simulink model "Detailed_PMSG_one_machine_GE"  (R2015b)
settings: Solver=VariableStepAuto  StartTime=0.0  StopTime=45  FixedStep=Ts  MaxStep=Ts  RelTol=1e-3
PreLoadFcn:
  | Ts=5e-6;
InitFcn:
  | Ts=5e-6;
undefined symbols (not defined in the file or in its folder): DiscIntNeverNeededParam, level
libraries: powerlib_extras x37, powerlib x16, simulink_extras x4, simulink x4
(part 1 of 2)
Description:
  | Copyright 2013-2015 Ruan Jiayang, Tsinghua Univ.
settings Model: Creator=XiaoLei  LastModifiedBy=Eren
settings DataIOCC: InitialState=xInit  SaveFinalState=on  SaveFormat=StructureWithTime  SignalLoggingSaveFormat=ModelDataLogs  SaveOutput=off  SignalLogging=off  SaveTime=off
settings OptimizationCC: ExpressionDepthLimit=2147483647  InitFltsAndDblsToZero=on
settings DebuggingCC: SaveWithParameterizedLinksMsg=none  UnderspecifiedInitializationDetection=Classic  MergeDetectMultiDrivingBlocksExec=none  SignalResolutionControl=TryResolveAllWithWarning  SolverPrmCheckMsg=warning  MultiTaskDSMMsg=warning  MultiTaskCondExecSysMsg=none  FcnCallInpInsideContextMsg=UseLocalSettings  UnconnectedInputMsg=none  UnconnectedOutputMsg=none  UnconnectedLineMsg=none  StateNameClashWarn=warning
settings HardwareCC: ProdBitPerPointer=32  ProdLargestAtomicFloat=None  ProdIntDivRoundTo=Undefined  ProdEndianess=Unspecified  ProdWordSize=32  ProdHWDeviceType=32-bit Generic
settings GRTTargetCC: TargetFcnLib=ansi_tfl_tmw.mat  GeneratePreprocessorConditionals=Disable all  CombineOutputUpdateFcns=off  GRTInterface=on
settings ConfigComp: CovModelRefEnable=Off

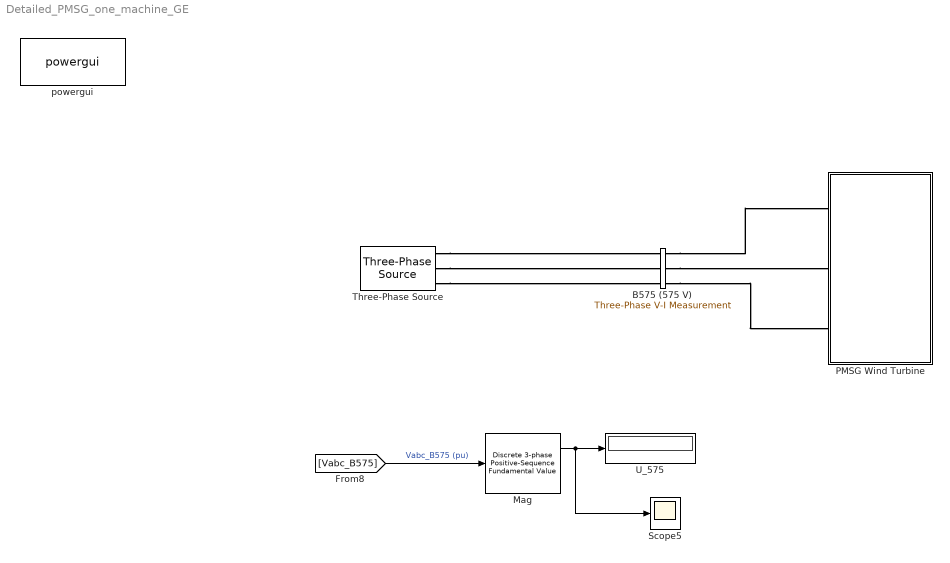
== system Detailed_PMSG_one_machine_GE ==
  B575 (575 V) : powerlib/Measurements/Three-Phase V-I Measurement  VoltageMeasurement=phase-to-ground  SetLabelV=on  LabelV=Vabc_B575  Vpu=on  VpuLL=off  CurrentMeasurement=yes  SetLabelI=on  LabelI=Iabc_B575  Ipu=on  Pbase=1.5e6  Vbase=575  OutputType=Complex  PhasorSimulation=off  PSBequivalent=0
  Mag : powerlib_extras/Discrete Measurements/Discrete 3-phase Positive-Sequence Fundamental Value  Freq=60  Par_Init=[0 0]  Ts=Ts
  PMSG Wind Turbine : Subsystem  mask{Vnom=575, Pnom=2.75e6, Fnom=50, RL_grid=[0.003 0.3], Vdc_nom=1150, Np=2, Fb_time_const=0.005}
      mask prompts: Vnom "Rated L-L Voltage(V)"; Pnom "Rated Power(VA)"; Fnom "Rated Frequency(Hz)"; RL_grid "Grid-side coupling impedance(p.u.)"; Vdc_nom "DC capacitor voltage(V)"; Np "Number of pole pairs"; Fb_time_const "Feed back time constant(s)"
      mask init:
      | R_RL=RL_grid(1);
      | L_RL=RL_grid(2);
  Scope5 : Scope
  Three-Phase Source : powerlib/Electrical Sources/Three-Phase Source  InternalConnection=Yg  VoltagePhases=off  Voltage=575  PhaseAngle=0  Voltage_phases=[25e3 25e3 25e3]/sqrt(3)  PhaseAngles_phases=[0 -120 +120]  Frequency=50  NonIdealSource=on  SpecifyImpedance=off  Resistance=0.0001  Inductance=16.58e-6  ShortCircuitLevel=100e6  BaseVoltage=575  XRratio=7  BusType=swing  Pref=10e3  Qref=0  Prefabc=[10e3, 10e3, 10e3]  Qrefabc=[0, 0, 0]  Qmin=-inf  Qmax=inf
  U_575 : Display
      settings: Decimation=10000
  powergui : powerlib/powergui  SimulationMode=Discrete  SolverType=Tustin/Backward Euler (TBE)  SampleTime=Ts  frequency=50  SPID=off  DisableSnubberDevices=off  DisableRonSwitches=off  DisableVfSwitches=off  SwTol=0  DisplayEquations=off  Interpol=off  ExternalGateDelay=off  methode=off  Ts=0  FunctionMessages=off  echomessages=off  HookPort=off  EnableUseOfTLC=off  x0status=blocks  frequencyindice=0  Pbase=100e6  ErrMax=1e-4  Iterations=50  UnitsV=kV  UnitsW=MW  buscounter=0  RestoreLinks=warning  ResistiveCurrentMeasurement=off  Frange=[0:2:500]  Ylog=off  Xlog=on  ShowGrid=off  save=off  variable=ZData  structure=0  ZoomFFT=on  StartTime=0.0  cycles=1  DisplayStyle=1  fundamental=60  FreqAxis=off  MaxFrequency=1000  frequencyindicesteady=1  RmsSteady=1  display=off
  wires:
  [Vabc_B575] -> Mag/1  "Vabc_B575 (pu)"
  Mag/1 -> U_575/1, Scope5/1
  connections:
  B575 (575 V)/RConn1 -- PMSG Wind Turbine/RConn1
  B575 (575 V)/RConn2 -- PMSG Wind Turbine/RConn2
  B575 (575 V)/RConn3 -- PMSG Wind Turbine/RConn3
  Three-Phase Source/RConn1 -- B575 (575 V)/LConn1
  Three-Phase Source/RConn2 -- B575 (575 V)/LConn2
  Three-Phase Source/RConn3 -- B575 (575 V)/LConn3

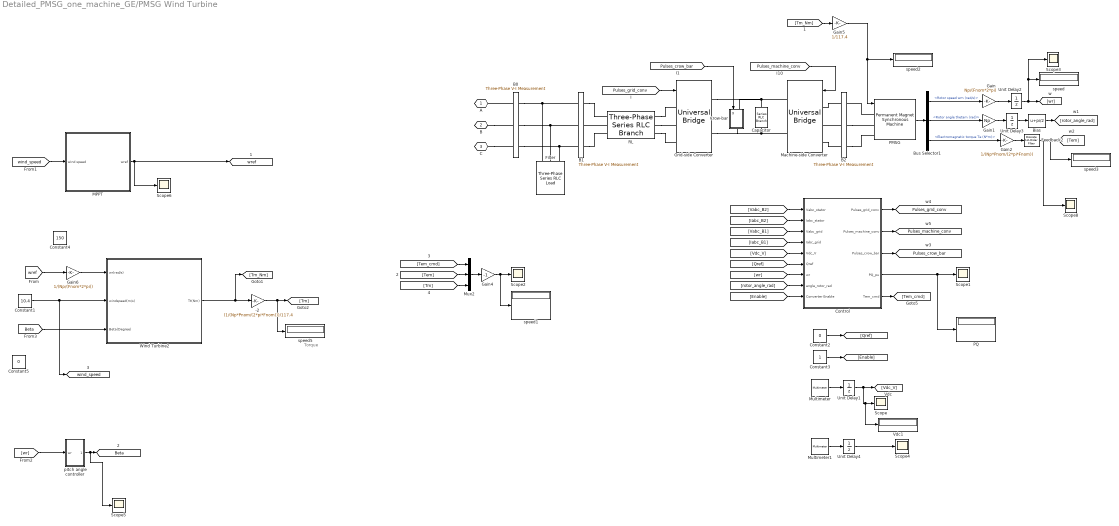
== system Detailed_PMSG_one_machine_GE/PMSG Wind Turbine ==
  note: Torque
  -2 : Gain  Gain=(1/(Np*Pnom/(2*pi*Fnom)))/117.4
  B0 : powerlib/Measurements/Three-Phase V-I Measurement  VoltageMeasurement=phase-to-ground  SetLabelV=on  LabelV=Vabc_B0  Vpu=on  VpuLL=off  CurrentMeasurement=yes  SetLabelI=on  LabelI=Iabc_B0  Ipu=on  Pbase=Pnom  Vbase=Vnom  OutputType=Complex  PhasorSimulation=off  PSBequivalent=0
  B1 : powerlib/Measurements/Three-Phase V-I Measurement  VoltageMeasurement=phase-to-ground  SetLabelV=on  LabelV=Vabc_B1  Vpu=on  VpuLL=off  CurrentMeasurement=yes  SetLabelI=on  LabelI=Iabc_B1  Ipu=on  Pbase=Pnom  Vbase=Vnom  OutputType=Complex  PhasorSimulation=off  PSBequivalent=0
  B2 : powerlib/Measurements/Three-Phase V-I Measurement  VoltageMeasurement=phase-to-ground  SetLabelV=on  LabelV=Vabc_B2  Vpu=on  VpuLL=off  CurrentMeasurement=yes  SetLabelI=on  LabelI=Iabc_B2  Ipu=on  Pbase=Pnom  Vbase=Vnom  OutputType=Complex  PhasorSimulation=off  PSBequivalent=0
  Bias : Bias  Bias=pi/2
  Bus Selector1 : BusSelector  OutputSignals=Rotor speed wm (rad/s),Rotor angle thetam (rad),Electromagnetic torque Te (N*m)
  Capacitor : powerlib/Elements/Series RLC Branch  LConnTagsString=__new0  RConnTagsString=__new0  BranchType=C  Resistance=1e-5  Inductance=1e-3  SetiL0=off  InitialCurrent=0  Capacitance=10000e-6  Setx0=on  InitialVoltage=Vdc_nom  Measurements=Branch voltage
  Constant1 : Constant  Value=10.4  SampleTime=Ts
  Constant2 : Constant  Value=0  SampleTime=Ts
  Constant3 : Constant  SampleTime=Ts
  Constant4 : Constant  Value=150  SampleTime=Ts
  Constant5 : Constant  Value=0  SampleTime=Ts
  Control : Subsystem
  Crow-bar : Subsystem
  Feedback2 : powerlib_extras/Discrete  Control Blocks/Discrete 1st-Order Filter  FilterType=Lowpass  Tc=0.3  Ts=Ts  Initialize=on  Vac_Init=[0 -25 60]  Vdc_Init=0  PlotResponse=off  param1=[1 500 0.1]
  Filter : powerlib/Elements/Three-Phase Series RLC Load  LConnTagsString=A|B|C  Configuration=Y (grounded)  NominalVoltage=Vnom  Vabc=[1e3 1e3 1e3]  Vabcp=[1e3 1e3 1e3]  NominalFrequency=Pnom  UnbalancedPower=off  ActivePower=0.005e6  InductivePower=0  CapacitivePower=0.04e6  Pabc=[10e3 9e3 11e3]  QLabc=[100 90 110]  QCabc=[100 90 110]  Pabcp=[10e3 9e3 11e3]  QLabcp=[100 90 110]  QCabcp=[100 90 110]  Measurements=None  LoadType=constant Z
  Gain : Gain  Gain=Np/(Fnom*2*pi)
  Gain1 : Gain  Gain=Np
  Gain2 : Gain  Gain=1/(Np*Pnom/(2*pi*Fnom))
  Gain4 : Gain  Gain=-1
  Gain5 : Gain  Gain=1/117.4
  Gain6 : Gain  Gain=1/(Np/(Fnom*2*pi))
  Grid-side Converter : powerlib/Power Electronics/Universal Bridge  Arms=3  SnubberResistance=1e5  SnubberCapacitance=inf  Device=IGBT / Diodes  Ron=1e-5  Lon=0  ForwardVoltages="[  0  0  ]"  ForwardVoltage=0  GTOparameters=[ 10e-6 , 20e-6 ]  IGBTparameters=[0 , 0]  Measurements=None  Measurements_2=None  converterType=Rectifier
  MPPT : Subsystem
  Machine-side Converter : powerlib/Power Electronics/Universal Bridge  Arms=3  SnubberResistance=1e5  SnubberCapacitance=inf  Device=IGBT / Diodes  Ron=1e-5  Lon=0  ForwardVoltages="[  0  0  ]"  ForwardVoltage=0  GTOparameters=[ 10e-6 , 20e-6 ]  IGBTparameters=[0 , 0]  Measurements=None  Measurements_2=None  converterType=Rectifier
  Multimeter : powerlib/Measurements/Multimeter  PhasorSimulation=off  OutputType=Complex  sel=1  L=2  Gain=1  yselected={'Ub: PMSG Wind Turbine/Capacitor'};  PSBOutputType=1  PSBequivalent=0  AxesSetting=[0,0.1,-100,100]  Display=0  SavedBlockNames=-11
  Multimeter1 : powerlib/Measurements/Multimeter  PhasorSimulation=off  OutputType=Complex  sel=2  L=2  Gain=1  yselected={'Ib: PMSG Wind Turbine/Crow-bar/R'};  PSBOutputType=1  PSBequivalent=0  AxesSetting=[0,0.1,-100,100]  Display=0  SavedBlockNames=-11
  Mux2 : Mux  Inputs=3
  PMSG : powerlib/Machines/Permanent Magnet Synchronous Machine  NbPhases=3  FluxDistribution=Sinusoidal  RotorType=Salient-pole  MechanicalLoad=Torque Tm  PresetModel=No  ShowDetailedParameters=on  MeasurementBus=off  Resistance=0.006  Inductance=8.5e-3  dqInductances="[2.48282e-4  2.92845e-4]"  La=2.48  MachineConstant=Flux linkage established by magnets (V.s)  Flux=4  VoltageCst=1451.0395  TorqueCst=12  Flat=120  Mechanical=[1088 0.01 Np]  PolePairs=Np  InitialConditions=[100,0, 0,0]  InitialConditions5ph=[0 0 0 0 0 0]  TsPowergui=0  TsBlock=Ts  RefAngle=90 degrees behind phase A axis (modified Park)
  PQ : Display
      settings: Decimation=10000
  RL : powerlib/Elements/Three-Phase Series RLC Branch  LConnTagsString=A|B|C  RConnTagsString=A|B|C  BranchType=RL  Resistance=R_RL*Vnom^2/Pnom  Inductance=L_RL*Vnom^2/Pnom/(2*pi*Fnom)  Capacitance=1.0  Measurements=None
  Scope{,1..6,8} (8 alike) : Scope
  Unit Delay{1..4} (4 alike) : UnitDelay  SampleTime=Ts
  Vdc1 : Display
      settings: Decimation=10000
  Wind Turbine2 : Subsystem
  pitch angle controller : Subsystem
  speed{,1..3,5} (5 alike) : Display
      speed settings: Decimation=10000
      speed1 settings: Decimation=10000
      speed2 settings: Decimation=1000
      speed3 settings: Decimation=1000
      speed5 settings: Decimation=1000
  A : PMIOPort  Tag=PMCPort  Port=1  Side=Right
  B : PMIOPort  Tag=PMCPort  Port=2  Side=Right
  C : PMIOPort  Tag=PMCPort  Port=3  Side=Right
  tag scope: Beta=global, Pulses_crow_bar=global, Pulses_grid_conv=global, Pulses_machine_conv=global, wind_speed=global, wref=global
  wires:
  Unit Delay1/1 -> [Vdc_V], Scope/1, Vdc1/1
  PMSG/1 -> Bus Selector1/1
  Bus Selector1/1 -> Gain/1  "<Rotor speed wm (rad/s)>"
  Gain/1 -> Unit Delay2/1
  Gain1/1 -> Unit Delay3/1
  Bus Selector1/2 -> Gain1/1  "<Rotor angle thetam (rad)>"
  Unit Delay2/1 -> [wr], speed/1, Scope3/1
  [Qref] -> Control/6(Qref)
  [Vdc_V] -> Control/5(Vdc_V)
  [Iabc_B1] -> Control/4(Iabc_grid)
  [Vabc_B1] -> Control/3(Vabc_grid)
  [Vabc_B2] -> Control/1(Vabc_stator)
  [Iabc_B2] -> Control/2(Iabc_stator)
  [Enable] -> Control/9(Converter Enable)
  Constant3/1 -> [Enable]
  Constant2/1 -> [Qref]
  [Pulses_grid_conv] -> Grid-side Converter/1
  [Pulses_machine_conv] -> Machine-side Converter/1
  Control/1(Pulses_grid_conv) -> [Pulses_grid_conv]
  Control/4(PQ_pu) -> Scope1/1, PQ/1
  Control/2(Pulses_machine_conv) -> [Pulses_machine_conv]
  [wr] -> Control/7(wr)
  [rotor_angle_rad] -> Control/8(angle_rotor_rad)
  Bus Selector1/3 -> Gain2/1  "<Electromagnetic torque Te (N*m)>"
  Bias/1 -> [rotor_angle_rad]
  Unit Delay3/1 -> Bias/1
  [Tm_Nm] -> Gain5/1
  Gain2/1 -> Feedback2/1
  Feedback2/1 -> Scope8/1, [Tem], speed3/1
  Control/5(Tem_cmd) -> [Tem_cmd]
  [Tem] -> Mux2/2
  [Tem_cmd] -> Mux2/1
  [Tm] -> Mux2/3
  Mux2/1 -> Gain4/1
  Gain4/1 -> Scope2/1, speed1/1
  Multimeter/1 -> Unit Delay1/1
  Control/3(Pulses_crow_bar) -> [Pulses_crow_bar]
  Unit Delay4/1 -> Scope4/1
  Multimeter1/1 -> Unit Delay4/1
  [Pulses_crow_bar] -> Crow-bar/1(g)
  [wr] -> pitch angle controller/1(wr)
  pitch angle controller/1(Beta) -> Scope5/1, [Beta]
  [wind_speed] -> MPPT/1(wind speed)
  MPPT/1("wref ") -> [wref], Scope6/1
  Gain5/1 -> speed2/1, PMSG/1
  -2/1 -> speed5/1, [Tm]
  Wind Turbine2/1(Tt(Nm)) -> [Tm_Nm], -2/1
  Constant1/1 -> [wind_speed], Wind Turbine2/2(windspeed(m/s))
  [wref] -> Gain6/1
  [Beta] -> Wind Turbine2/3(Beta(Degree))
  Gain6/1 -> Wind Turbine2/1(wr(rad/s))
  connections:
  RL/RConn1 -- Grid-side Converter/LConn1
  RL/RConn2 -- Grid-side Converter/LConn2
  RL/RConn3 -- Grid-side Converter/LConn3
  B1/LConn1 -- Filter/LConn1 -- B0/RConn1
  B1/LConn2 -- Filter/LConn2 -- B0/RConn2
  B1/LConn3 -- Filter/LConn3 -- B0/RConn3
  B1/RConn1 -- RL/LConn1
  RL/LConn2 -- B1/RConn2
  B1/RConn3 -- RL/LConn3
  B2/RConn2 -- PMSG/LConn2
  PMSG/LConn1 -- B2/RConn1
  B2/LConn1 -- Machine-side Converter/LConn1
  Machine-side Converter/LConn3 -- B2/LConn3
  B2/LConn2 -- Machine-side Converter/LConn2
  B0/LConn1 -- A/RConn1
  B/RConn1 -- B0/LConn2
  C/RConn1 -- B0/LConn3
  B2/RConn3 -- PMSG/LConn3
  Grid-side Converter/RConn1 -- Crow-bar/LConn1 -- Machine-side Converter/RConn1 -- Capacitor/LConn1
  Grid-side Converter/RConn2 -- Crow-bar/RConn1 -- Machine-side Converter/RConn2 -- Capacitor/RConn1

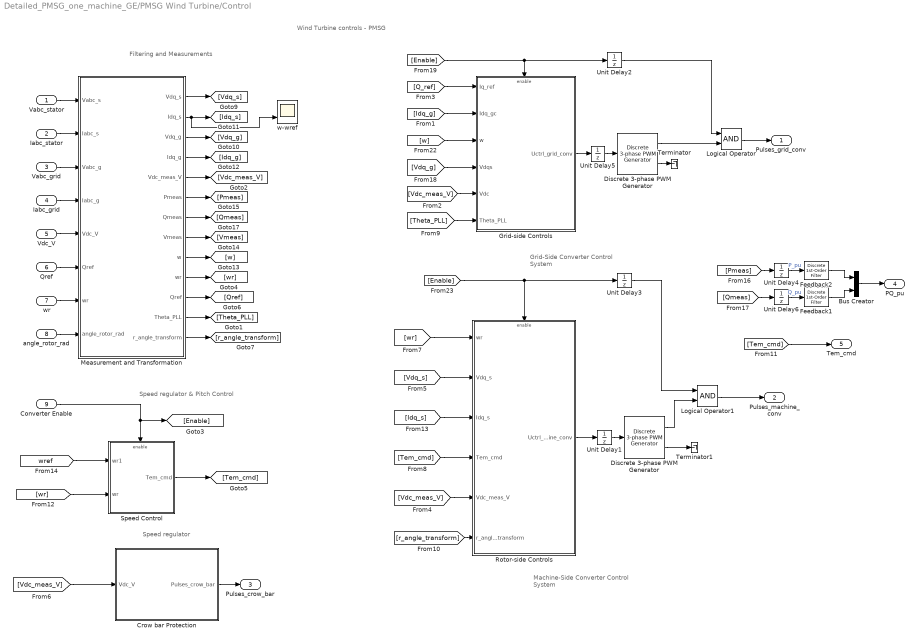
== system Detailed_PMSG_one_machine_GE/PMSG Wind Turbine/Control ==
  note: Wind Turbine controls - PMSG
  note: Filtering and
      | Measurements
  note: Speed regulator & Pitch Control
  note: Speed regulator
  note: Grid-Side Converter
      | Control System
  note: Machine-Side Converter
      | Control System
  Vabc_stator : Inport
  Iabc_stator : Inport  Port=2
  Vabc_grid : Inport  Port=3
  Iabc_grid : Inport  Port=4
  Vdc_V : Inport  Port=5
  Qref : Inport  Port=6
  wr : Inport  Port=7
  angle_rotor_rad : Inport  Port=8
  Converter Enable : Inport  Port=9
  Bus Creator : BusCreator  Inputs=2
  Crow bar Protection : Subsystem
  Discrete 3-phase PWM Generator : powerlib_extras/Discrete  Control Blocks/Discrete 3-phase PWM Generator  ModulatorType=2-level  ModulatorMode=Un-synchronized  nF=27  Fc=2250  ModulatingSignals=off  m=0.2  Freq=60  Phase=0  Ts=Ts
  "Discrete 3-phase PWM Generator " : powerlib_extras/Discrete  Control Blocks/Discrete 3-phase PWM Generator  ModulatorType=2-level  ModulatorMode=Un-synchronized  nF=27  Fc=3000  ModulatingSignals=off  m=0.2  Freq=60  Phase=0  Ts=Ts
  Feedback1 : powerlib_extras/Discrete  Control Blocks/Discrete 1st-Order Filter  FilterType=Lowpass  Tc=0.3  Ts=Ts  Initialize=on  Vac_Init=[0 -25 50]  Vdc_Init=0  PlotResponse=off  param1=[1 500 0.1]
  Feedback2 : powerlib_extras/Discrete  Control Blocks/Discrete 1st-Order Filter  FilterType=Lowpass  Tc=0.3  Ts=Ts  Initialize=on  Vac_Init=[0 -25 50]  Vdc_Init=0  PlotResponse=off  param1=[1 500 0.1]
  Grid-side Controls : Subsystem
  Logical Operator : Logic  AllPortsSameDT=off  OutDataTypeStr=boolean
  Logical Operator1 : Logic  AllPortsSameDT=off  OutDataTypeStr=boolean
  Measurement and Transformation : Subsystem
  Rotor-side Controls : Subsystem
  Speed Control : Subsystem
  Terminator : Terminator
  Terminator1 : Terminator
  Unit Delay{1..6} (6 alike) : UnitDelay  SampleTime=Ts
  w-wref : Scope  NumInputPorts=2
  Pulses_grid_conv : Outport
  Pulses_machine_conv : Outport  Port=2
  Pulses_crow_bar : Outport  Port=3
  PQ_pu : Outport  Port=4
  Tem_cmd : Outport  Port=5
  wires:
  [Pmeas] -> Unit Delay4/1
  [Qmeas] -> Unit Delay6/1
  wr/1 -> Measurement and Transformation/7(wr)
  Qref/1 -> Measurement and Transformation/6(Qref)
  Vdc_V/1 -> Measurement and Transformation/5(Vdc_V)
  Measurement and Transformation/11("Qref ") -> [Qref]
  Measurement and Transformation/10("wr ") -> [wr]
  Measurement and Transformation/5(Vdc_meas_V) -> [Vdc_meas_V]
  Measurement and Transformation/9(w) -> [w]
  Measurement and Transformation/6(Pmeas) -> [Pmeas]
  Measurement and Transformation/4(Idq_g) -> [Idq_g]
  Measurement and Transformation/3(Vdq_g) -> [Vdq_g]
  Measurement and Transformation/2(Idq_s) -> w-wref/2, [Idq_s]
  angle_rotor_rad/1 -> Measurement and Transformation/8(angle_rotor_rad)
  Iabc_stator/1 -> Measurement and Transformation/2(Iabc_s)
  Iabc_grid/1 -> Measurement and Transformation/4(Iabc_g)
  Vabc_grid/1 -> Measurement and Transformation/3(Vabc_g)
  Vabc_stator/1 -> Measurement and Transformation/1(Vabc_s)
  Measurement and Transformation/7(Qmeas) -> [Qmeas]
  Measurement and Transformation/8(Vmeas) -> [Vmeas]
  Measurement and Transformation/12(Theta_PLL) -> [Theta_PLL]
  Measurement and Transformation/13(r_angle_transform) -> [r_angle_transform]
  Speed Control/1(Tem_cmd) -> [Tem_cmd]
  [wr] -> Speed Control/2(wr)
  Converter Enable/1 -> Speed Control/Enable, [Enable]
  [Tem_cmd] -> Tem_cmd/1
  Measurement and Transformation/1(Vdq_s) -> [Vdq_s]
  Grid-side Controls/1(Uctrl_grid_conv) -> Unit Delay5/1
  Discrete 3-phase PWM Generator/2 -> Terminator/1
  Unit Delay5/1 -> Discrete 3-phase PWM Generator/1
  [Vdc_meas_V] -> Grid-side Controls/5(Vdc)
  [Vdq_g] -> Grid-side Controls/4(Vdqs)
  [w] -> Grid-side Controls/3(w)
  [Idq_g] -> Grid-side Controls/2(Idq_gc)
  [Q_ref] -> Grid-side Controls/1(Iq_ref)
  [Theta_PLL] -> Grid-side Controls/6(Theta_PLL)
  [Enable] -> Grid-side Controls/Enable, Unit Delay2/1
  Logical Operator/1 -> Pulses_grid_conv/1
  Discrete 3-phase PWM Generator/1 -> Logical Operator/2
  Unit Delay2/1 -> Logical Operator/1
  "Discrete 3-phase PWM Generator "/2 -> Terminator1/1
  Unit Delay1/1 -> "Discrete 3-phase PWM Generator "/1
  [Enable] -> Unit Delay3/1, Rotor-side Controls/Enable
  Logical Operator1/1 -> Pulses_machine_conv/1
  "Discrete 3-phase PWM Generator "/1 -> Logical Operator1/2
  Unit Delay3/1 -> Logical Operator1/1
  [wr] -> Rotor-side Controls/1(wr)
  [Vdc_meas_V] -> Rotor-side Controls/5(Vdc_meas_V)
  [r_angle_transform] -> Rotor-side Controls/6(r_angle_transform)
  [Vdq_s] -> Rotor-side Controls/2(" Vdq_s")
  [Idq_s] -> Rotor-side Controls/3(Idq_s)
  Rotor-side Controls/1(Uctrl_machine_conv) -> Unit Delay1/1
  [Tem_cmd] -> Rotor-side Controls/4(Tem_cmd)
  Unit Delay4/1 -> Feedback2/1  "P_pu"
  Feedback2/1 -> Bus Creator/1
  Unit Delay6/1 -> Feedback1/1  "Q_pu"
  Feedback1/1 -> Bus Creator/2
  Crow bar Protection/1(Pulses_crow_bar) -> Pulses_crow_bar/1
  [Vdc_meas_V] -> Crow bar Protection/1(Vdc_V)
  Bus Creator/1 -> PQ_pu/1
  [wref] -> Speed Control/1(wr1)

== system Detailed_PMSG_one_machine_GE/PMSG Wind Turbine/Crow-bar ==
  g : Inport
  IGBT : powerlib/Power Electronics/IGBT//Diode  Ron=1e-5  Rs=1e5  Cs=inf  Measurements=off
  R : powerlib/Elements/Series RLC Branch  LConnTagsString=__new0  RConnTagsString=__new0  BranchType=R  Resistance=1  Inductance=1e-3  SetiL0=off  InitialCurrent=0  Capacitance=1e-6  Setx0=off  InitialVoltage=0  Measurements=Branch current
  + : PMIOPort  Port=1  Side=Left
  - : PMIOPort  Port=2  Side=Right
  wires:
  g/1 -> IGBT/1
  connections:
  R/LConn1 -- IGBT/RConn1
  +/RConn1 -- IGBT/LConn1
  -/RConn1 -- R/RConn1

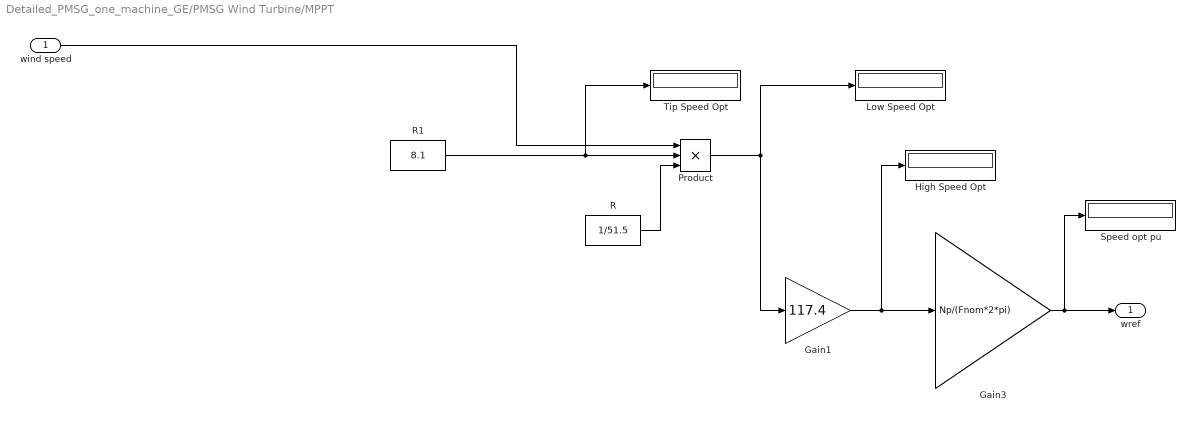
== system Detailed_PMSG_one_machine_GE/PMSG Wind Turbine/MPPT ==
  wind speed : Inport
  " High Speed Opt " : Display
  " Speed opt pu " : Display
  Gain1 : Gain  Gain=117.4
  Gain3 : Gain  Gain=Np/(Fnom*2*pi)
  "Low Speed Opt " : Display
  Product : Product  Inputs=3
  R : Constant  Value=1/51.5
  R1 : Constant  Value=8.1
  "Tip Speed Opt " : Display
  "wref " : Outport
  wires:
  R1/1 -> "Tip Speed Opt "/1, Product/2
  R/1 -> Product/3
  wind speed/1 -> Product/1
  Product/1 -> "Low Speed Opt "/1, Gain1/1
  Gain3/1 -> " Speed opt pu "/1, "wref "/1
  Gain1/1 -> " High Speed Opt "/1, Gain3/1

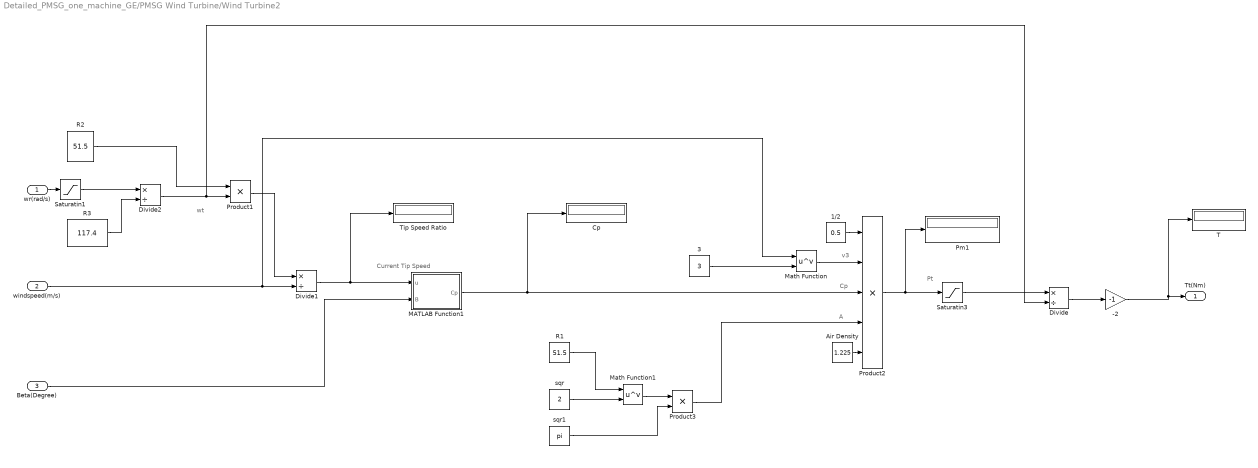
== system Detailed_PMSG_one_machine_GE/PMSG Wind Turbine/Wind Turbine2 ==
  note: Pt
  note: v3
  note: Cp
  note: A
  note: wt
  note: Current Tip Speed
  wr(rad/s) : Inport
  windspeed(m/s) : Inport  Port=2
  Beta(Degree) : Inport  Port=3
  -2 : Gain  Gain=-1
  1/2 : Constant  Value=0.5
  3 : Constant  Value=3
  Air Density : Constant  Value=1.225
  Cp : Display
  Divide : Product  Inputs=*/
  Divide1 : Product  Inputs=*/
  Divide2 : Product  Inputs=*/
  MATLAB Function1 : MATLAB Function  TreatAsAtomicUnit=on
  Math Function : Math  Operator=pow  SaturateOnIntegerOverflow=on
  Math Function1 : Math  Operator=pow  SaturateOnIntegerOverflow=on
  Pm1 : Display
  Product1 : Product
  Product2 : Product  Inputs=5
  Product3 : Product
  R1 : Constant  Value=51.5
  R2 : Constant  Value=51.5
  R3 : Constant  Value=117.4
  Saturatin1 : Saturate  UpperLimit=inf  LowerLimit=1e-8
  Saturatin3 : Saturate  UpperLimit=2.75e6  LowerLimit=1e-6
  T : Display
  "Tip Speed Ratio " : Display
  sqr : Constant  Value=2
  sqr1 : Constant  Value=pi
  Tt(Nm) : Outport
  wires:
  Air Density/1 -> Product2/5
  1/2/1 -> Product2/1
  Product3/1 -> Product2/4
  Math Function1/1 -> Product3/1
  sqr1/1 -> Product3/2
  Math Function/1 -> Product2/2
  sqr/1 -> Math Function1/2
  R1/1 -> Math Function1/1
  Product2/1 -> Saturatin3/1, Pm1/1
  3/1 -> Math Function/2
  R2/1 -> Product1/1
  wr(rad/s)/1 -> Saturatin1/1
  Product1/1 -> Divide1/1
  Divide1/1 -> MATLAB Function1/1(u), "Tip Speed Ratio "/1
  Divide2/1 -> Divide/2, Product1/2
  MATLAB Function1/1(Cp) -> Product2/3, Cp/1
  R3/1 -> Divide2/2
  windspeed(m/s)/1 -> Math Function/1, Divide1/2
  Beta(Degree)/1 -> MATLAB Function1/2(B)
  Divide/1 -> -2/1
  Saturatin3/1 -> Divide/1
  Saturatin1/1 -> Divide2/1
  -2/1 -> T/1, Tt(Nm)/1

== system Detailed_PMSG_one_machine_GE/PMSG Wind Turbine/pitch angle controller ==
  wr : Inport
  Constant1 : Constant  Value=1735/1500  SampleTime=Ts
  pitch angle controller : Subsystem
  Beta : Outport
  wires:
  Constant1/1 -> pitch angle controller/2(Ref)
  pitch angle controller/1(pitch) -> Beta/1
  wr/1 -> pitch angle controller/1(wg)

== system Detailed_PMSG_one_machine_GE/PMSG Wind Turbine/Control/Crow bar Protection ==
  Vdc_V : Inport
  Relay : Relay  OnSwitchValue=1500  OffSwitchValue=1300
  Pulses_crow_bar : Outport
  wires:
  Vdc_V/1 -> Relay/1
  Relay/1 -> Pulses_crow_bar/1

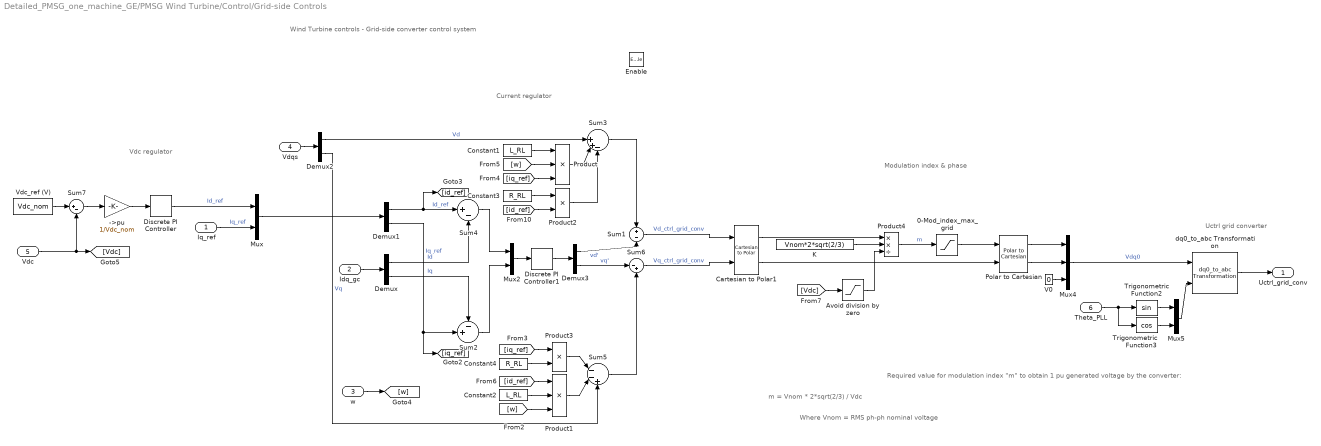
== system Detailed_PMSG_one_machine_GE/PMSG Wind Turbine/Control/Grid-side Controls ==
  note: Wind Turbine controls - Grid-side converter control system
  note: Where Vnom = RMS ph-ph nominal voltage
  note: m = Vnom * 2*sqrt(2/3) / Vdc
  note: Required value for modulation index "m" to obtain 1 pu generated voltage by the converter:
  note: Vdc regulator
  note: Current regulator
  note: Modulation index & phase
  note: Uctrl grid converter
  Iq_ref : Inport
  Idq_gc : Inport  Port=2
  w : Inport  Port=3
  Vdqs : Inport  Port=4
  Vdc : Inport  Port=5
  Theta_PLL : Inport  Port=6
  Enable : EnablePort
  ->pu : Gain  Gain=1/Vdc_nom
  0-Mod_index_max_grid : Saturate  UpperLimit=1.1  LowerLimit=0
  Avoid division by zero : Saturate  UpperLimit=inf  LowerLimit=1e-6
  Cartesian to Polar1 : simulink_extras/Transformations/Cartesian to Polar
  Constant1 : Constant  Value=L_RL
  Constant2 : Constant  Value=L_RL
  Constant3 : Constant  Value=R_RL
  Constant4 : Constant  Value=R_RL
  Demux{,1..3} (4 alike) : Demux  Outputs=2
  Discrete PI Controller : powerlib_extras/Discrete  Control Blocks/Discrete PI Controller  Kp=8  Ki=400  Par_Limits=[1 -1]*1.2  Init=0  Ts=Ts
  Discrete PI Controller1 : powerlib_extras/Discrete  Control Blocks/Discrete PI Controller  Kp=0.83  Ki=5  Par_Limits=[1.0 -1.0] *1.1  Init=0  Ts=Ts
  K : Constant  Value=Vnom*2*sqrt(2/3)
  Mux : Mux  Inputs=2
  Mux2 : Mux  Inputs=2
  Mux4 : Mux  Inputs=3
  Mux5 : Mux  Inputs=2
  Polar to Cartesian : simulink_extras/Transformations/Polar to Cartesian
  Product : Product  Inputs=3  SaturateOnIntegerOverflow=on  InputSameDT=on  OutDataTypeStr=Inherit: Same as first input
  Product1 : Product  Inputs=3  SaturateOnIntegerOverflow=on  InputSameDT=on  OutDataTypeStr=Inherit: Same as first input
  Product2 : Product  SaturateOnIntegerOverflow=on  InputSameDT=on  OutDataTypeStr=Inherit: Same as first input
  Product3 : Product  SaturateOnIntegerOverflow=on  InputSameDT=on  OutDataTypeStr=Inherit: Same as first input
  Product4 : Product  Inputs=**/  SaturateOnIntegerOverflow=on  InputSameDT=on  OutDataTypeStr=Inherit: Same as first input
  Sum1 : Sum  Inputs=+-  SaturateOnIntegerOverflow=on  InputSameDT=on  OutDataTypeStr=Inherit: Same as first input
  Sum2 : Sum  Inputs=-+|  SaturateOnIntegerOverflow=on  InputSameDT=on  OutDataTypeStr=Inherit: Same as first input
  Sum3 : Sum  Inputs=||++-  SaturateOnIntegerOverflow=on  InputSameDT=on  OutDataTypeStr=Inherit: Same as first input
  Sum4 : Sum  Inputs=|+-  SaturateOnIntegerOverflow=on  InputSameDT=on  OutDataTypeStr=Inherit: Same as first input
  Sum5 : Sum  Inputs=|--+  SaturateOnIntegerOverflow=on  InputSameDT=on  OutDataTypeStr=Inherit: Same as first input
  Sum6 : Sum  Inputs=|-+  SaturateOnIntegerOverflow=on  InputSameDT=on  OutDataTypeStr=Inherit: Same as first input
  Sum7 : Sum  Inputs=|+-  SaturateOnIntegerOverflow=on  InputSameDT=on  OutDataTypeStr=Inherit: Same as first input
  Trigonometric Function2 : Trigonometry
  Trigonometric Function3 : Trigonometry  Operator=cos
  V0 : Constant  Value=0
  Vdc_ref (V) : Constant  Value=Vdc_nom
  dq0_to_abc Transformation : powerlib_extras/Measurements/dq0_to_abc Transformation
  Uctrl_grid_conv : Outport
  wires:
  Vdc_ref (V)/1 -> Sum7/1
  Iq_ref/1 -> Mux/2  "Iq_ref"
  Vdc/1 -> Sum7/2, [Vdc]
  ->pu/1 -> Discrete PI Controller/1
  Sum7/1 -> ->pu/1
  Discrete PI Controller/1 -> Mux/1  "Id_ref"
  Sum5/1 -> Sum6/2
  Sum3/1 -> Sum1/1
  Demux1/1 -> [id_ref], Sum4/1  "Id_ref"
  Demux1/2 -> Sum2/2, [iq_ref]  "Iq_ref"
  Demux3/2 -> Sum6/1  "vq'"
  Demux3/1 -> Sum1/2  "vd'"
  [id_ref] -> Product1/1
  [iq_ref] -> Product3/1
  [id_ref] -> Product2/2
  [iq_ref] -> Product/3
  [w] -> Product/2
  [w] -> Product1/3
  Sum2/1 -> Mux2/2
  Sum4/1 -> Mux2/1
  Product3/1 -> Sum5/1
  Product2/1 -> Sum3/3
  Demux2/2 -> Sum5/3  "Vq"
  Product1/1 -> Sum5/2
  Constant4/1 -> Product3/2
  Constant3/1 -> Product2/1
  Product/1 -> Sum3/2
  Demux/1 -> Sum4/2  "Id"
  Demux/2 -> Sum2/1  "Iq"
  Vdqs/1 -> Demux2/1
  Constant1/1 -> Product/1
  Demux2/1 -> Sum3/1  "Vd"
  Mux2/1 -> Discrete PI Controller1/1
  Discrete PI Controller1/1 -> Demux3/1
  Constant2/1 -> Product1/2
  w/1 -> [w]
  Idq_gc/1 -> Demux/1
  Mux/1 -> Demux1/1
  Cartesian to Polar1/2 -> Polar to Cartesian/2
  0-Mod_index_max_grid/1 -> Polar to Cartesian/1
  Cartesian to Polar1/1 -> Product4/1
  Avoid division by zero/1 -> Product4/3
  K/1 -> Product4/2
  Product4/1 -> 0-Mod_index_max_grid/1  "m"
  [Vdc] -> Avoid division by zero/1
  Mux5/1 -> dq0_to_abc Transformation/2
  Trigonometric Function2/1 -> Mux5/1
  Trigonometric Function3/1 -> Mux5/2
  V0/1 -> Mux4/3
  Polar to Cartesian/1 -> Mux4/1
  Polar to Cartesian/2 -> Mux4/2
  Mux4/1 -> dq0_to_abc Transformation/1  "Vdq0"
  Theta_PLL/1 -> Trigonometric Function3/1, Trigonometric Function2/1
  dq0_to_abc Transformation/1 -> Uctrl_grid_conv/1
  Sum1/1 -> Cartesian to Polar1/1  "Vd_ctrl_grid_conv"
  Sum6/1 -> Cartesian to Polar1/2  "Vq_ctrl_grid_conv"

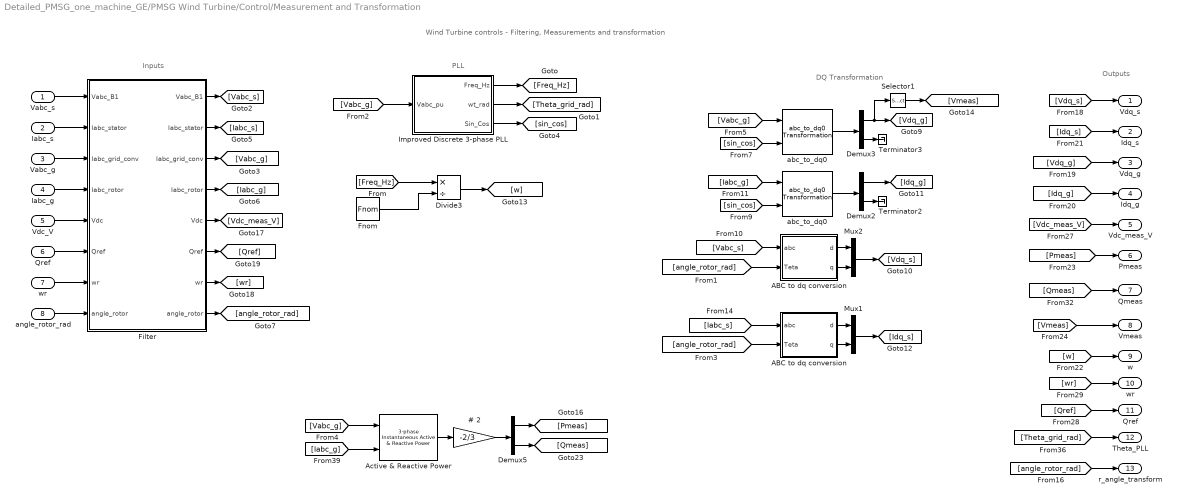
== system Detailed_PMSG_one_machine_GE/PMSG Wind Turbine/Control/Measurement and Transformation ==
  note: Wind Turbine controls - Filtering, Measurements and transformation
  note: Outputs
  note: Inputs
  note: PLL
  note: DQ Transformation
  Vabc_s : Inport
  Iabc_s : Inport  Port=2
  Vabc_g : Inport  Port=3
  Iabc_g : Inport  Port=4
  Vdc_V : Inport  Port=5
  Qref : Inport  Port=6
  wr : Inport  Port=7
  angle_rotor_rad : Inport  Port=8
  " Improved Discrete 3-phase PLL" : Subsystem  AncestorBlock=|  mask(Discrete 3-phase PLL){Fmin=0.75*Fnom, Par_Init=[0 Fnom], ParK=[5 3.2 1 50], Ts=Ts}
      | powerlib_extras/Discrete 
      | Control Blocks/Discrete
      | 3-phase PLL
      mask prompts: Fmin "Minimum frequency (Hz):"; Par_Init "Initial inputs:[ Phase(degrees)   Frequency(Hz) ]"; ParK "Regulator gains [ Kp1 Kp2  Ki1  Ki2 ]"; Ts "Sample time:"
      mask help:
      | This Phase Locked Loop (PLL) system can be used  to synchronize on a set of variable frequency, three-phase sinusoidal signals.
      |
      | Input 1: Vector containing the normalized
      |              three-phase signals [Va Vb Vc]
      | Output 1:  Measured frequency (Hz) = w/(2pi)
      | Output 2:  Ramp w.t   varying between  0 and 2*pi,
      | synchronized on zero crossings of the fundamental (positive-sequence) of phase A.
      | Output 3: Vector [sin(wt) cos(wt)]
      mask init:
      | Kp1=ParK(1);
      | Kp2=ParK(2);
      | Ki1=ParK(3);
      | Ki2=ParK(4);
      | Phase_Init=Par_Init(1);
      | Finit=Par_Init(2);
      | power_initmask();
      settings: OpenFcn=power_openblockproxy();
  # 2 : Gain  Gain=-2/3  SaturateOnIntegerOverflow=on  OutDataTypeStr=Inherit: Same as input  ParamDataTypeStr=Inherit: Same as input
  "ABC to dq conversion " : Subsystem
  ABC to dq conversion : Subsystem
  Active & Reactive Power : powerlib_extras/Measurements/3-phase  Instantaneous  Active & Reactive Power
  Demux2 : Demux  Outputs=[2 1]
  Demux3 : Demux  Outputs=[2 1]
  Demux5 : Demux  Outputs=2
  Divide3 : Product  Inputs=*/
  Filter : Subsystem  mask{Freq=1e4, Zeta1=0.707, Ts=Ts}
      mask prompts: Freq "Cut-off frequency (Hz):"; Zeta1 "Damping factor Zeta:"; Ts "Sample time"
  Fnom : Constant  Value=Fnom
  Mux1 : Mux  Inputs=2
  Mux2 : Mux  Inputs=2
  Selector1 : Selector  InputPortWidth=2  IndexOptions=Index vector (dialog)  Indices=1  OutputSizes=[(-2)]
  Terminator2 : Terminator
  Terminator3 : Terminator
  abc_to_dq0 : powerlib_extras/Measurements/abc_to_dq0 Transformation
  "abc_to_dq0 " : powerlib_extras/Measurements/abc_to_dq0 Transformation
  Vdq_s : Outport
  Idq_s : Outport  Port=2
  Vdq_g : Outport  Port=3
  Idq_g : Outport  Port=4
  Vdc_meas_V : Outport  Port=5
  Pmeas : Outport  Port=6
  Qmeas : Outport  Port=7
  Vmeas : Outport  Port=8
  w : Outport  Port=9
  "wr " : Outport  Port=10
  "Qref " : Outport  Port=11
  Theta_PLL : Outport  Port=12
  r_angle_transform : Outport  Port=13
  wires:
  angle_rotor_rad/1 -> Filter/8(angle_rotor)
  Filter/8("angle_rotor ") -> [angle_rotor_rad]
  Filter/7("wr ") -> [wr]
  Filter/6("Qref ") -> [Qref]
  Filter/5("Vdc ") -> [Vdc_meas_V]
  Filter/4("Iabc_rotor ") -> [Iabc_g]
  Filter/3("Iabc_grid_conv ") -> [Vabc_g]
  Filter/2("Iabc_stator ") -> [Iabc_s]
  Filter/1("Vabc_B1 ") -> [Vabc_s]
  [wr] -> "wr "/1
  [Qref] -> "Qref "/1
  [Vdc_meas_V] -> Vdc_meas_V/1
  wr/1 -> Filter/7(wr)
  Qref/1 -> Filter/6(Qref)
  Vdc_V/1 -> Filter/5(Vdc)
  Iabc_g/1 -> Filter/4(Iabc_rotor)
  Vabc_g/1 -> Filter/3(Iabc_grid_conv)
  Iabc_s/1 -> Filter/2(Iabc_stator)
  Vabc_s/1 -> Filter/1(Vabc_B1)
  [angle_rotor_rad] -> "ABC to dq conversion "/2(Teta)
  [Vmeas] -> Vmeas/1
  [Pmeas] -> Pmeas/1
  [w] -> w/1
  [Idq_s] -> Idq_s/1
  [Idq_g] -> Idq_g/1
  [Vdq_g] -> Vdq_g/1
  [Vdq_s] -> Vdq_s/1
  Demux2/1 -> [Idq_g]
  [Iabc_s] -> "ABC to dq conversion "/1(abc)
  [Iabc_g] -> "abc_to_dq0 "/1
  [Vabc_s] -> ABC to dq conversion/1(abc)
  [sin_cos] -> "abc_to_dq0 "/2
  [sin_cos] -> abc_to_dq0/2
  [Vabc_g] -> abc_to_dq0/1
  [Freq_Hz] -> Divide3/1
  Divide3/1 -> [w]
  Fnom/1 -> Divide3/2
  "abc_to_dq0 "/1 -> Demux2/1
  Demux2/2 -> Terminator2/1
  abc_to_dq0/1 -> Demux3/1
  Demux3/2 -> Terminator3/1
  Demux3/1 -> [Vdq_g], Selector1/1
  [Qmeas] -> Qmeas/1
  [Theta_grid_rad] -> Theta_PLL/1
  [angle_rotor_rad] -> r_angle_transform/1
  [Vabc_g] -> " Improved Discrete 3-phase PLL"/1(Vabc_pu)
  " Improved Discrete 3-phase PLL"/2(wt_rad) -> [Theta_grid_rad]
  " Improved Discrete 3-phase PLL"/3(Sin_Cos) -> [sin_cos]
  " Improved Discrete 3-phase PLL"/1(Freq_Hz) -> [Freq_Hz]
  [Vabc_g] -> Active & Reactive Power/1
  [Iabc_g] -> Active & Reactive Power/2
  Demux5/1 -> [Pmeas]
  Demux5/2 -> [Qmeas]
  Active & Reactive Power/1 -> # 2/1
  # 2/1 -> Demux5/1
  Selector1/1 -> [Vmeas]
  [angle_rotor_rad] -> ABC to dq conversion/2(Teta)
  ABC to dq conversion/1(d) -> Mux2/1
  ABC to dq conversion/2(q) -> Mux2/2
  Mux2/1 -> [Vdq_s]
  "ABC to dq conversion "/1(d) -> Mux1/1
  "ABC to dq conversion "/2(q) -> Mux1/2
  Mux1/1 -> [Idq_s]

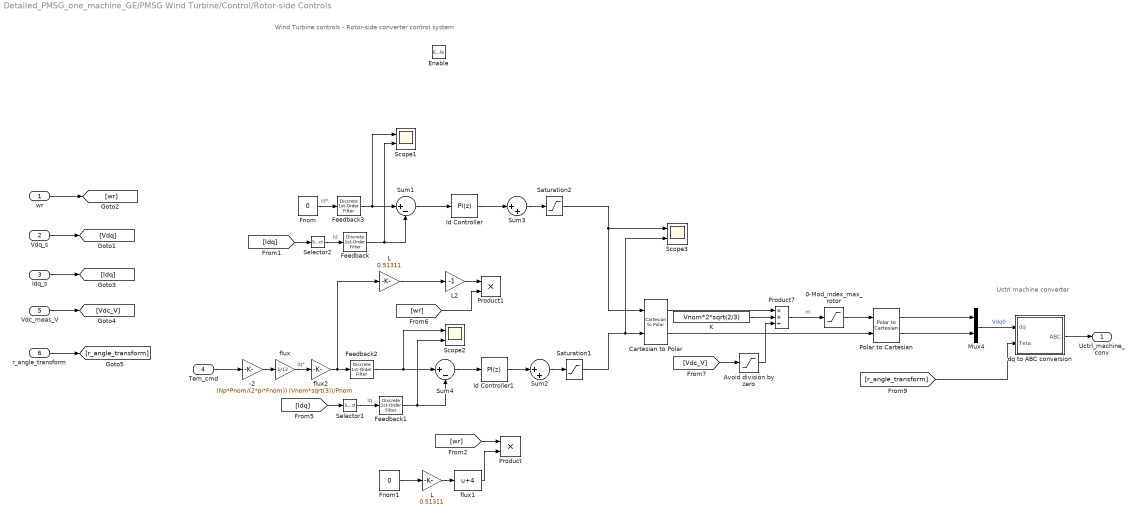
== system Detailed_PMSG_one_machine_GE/PMSG Wind Turbine/Control/Rotor-side Controls ==
  note: Wind Turbine controls - Rotor-side converter control system
  note: Uctrl machine converter
  wr : Inport
  " Vdq_s" : Inport  Port=2
  Idq_s : Inport  Port=3
  Tem_cmd : Inport  Port=4
  Vdc_meas_V : Inport  Port=5
  r_angle_transform : Inport  Port=6
  Enable : EnablePort
  -2 : Gain  Gain=(Np*Pnom/(2*pi*Fnom))
  0-Mod_index_max_rotor : Saturate  UpperLimit=2  LowerLimit=0
  Avoid division by zero : Saturate  UpperLimit=inf  LowerLimit=1e-6
  Cartesian to Polar : simulink_extras/Transformations/Cartesian to Polar
  Feedback{,1..3} (4 alike) : powerlib_extras/Discrete  Control Blocks/Discrete 1st-Order Filter  FilterType=Lowpass  Tc=Fb_time_const  Ts=Ts  Initialize=on  Vac_Init=[0 -25 50]  Vdc_Init=0  PlotResponse=off  param1=[1 500 0.1]
  Fnom : Constant  Value=0
  Fnom1 : Constant  Value=0
  Id Controller : simulink/Continuous/PID Controller  Controller=PI  TimeDomain=Discrete-time  SampleTime=Ts  IntegratorMethod=Forward Euler  FilterMethod=Forward Euler  Form=Parallel  UseFilter=on  ControllerParametersSource=internal  P=0.1  I=0.01  D=0  N=100  InitialConditionSource=internal  InitialConditionForIntegrator=0  InitialConditionForFilter=0  ExternalReset=none  ZeroCross=off  LimitOutput=off  UpperSaturationLimit=2  LowerSaturationLimit=-2  LinearizeAsGain=off  AntiWindupMode=clamping  Kb=1  TrackingMode=off  Kt=1  PParamMin=[]  PParamMax=[]  IParamMin=[]  IParamMax=[]  DParamMin=[]  DParamMax=[]  NParamMin=[]  NParamMax=[]  KbParamMin=[]  KbParamMax=[]  KtParamMin=[]  KtParamMax=[]  POutMin=[]  POutMax=[]  IOutMin=[]  IOutMax=[]  DOutMin=[]  DOutMax=[]  NOutMin=[]  NOutMax=[]  KbOutMin=[]  KbOutMax=[]  KtOutMin=[]  KtOutMax=[]  IntegratorOutMin=[]  IntegratorOutMax=[]  FilterOutMin=[]  FilterOutMax=[]  SumOutMin=[]  SumOutMax=[]  SumI1OutMin=[]  SumI1OutMax=[]  SumI2OutMin=[]  SumI2OutMax=[]  SumI3OutMin=[]  SumI3OutMax=[]  SumDOutMin=[]  SumDOutMax=[]  SaturationOutMin=[]  SaturationOutMax=[]  IntegratorContinuousStateAttributes=''  IntegratorStateMustResolveToSignalObject=off  IntegratorRTWStateStorageClass=Auto  FilterContinuousStateAttributes=''  FilterStateMustResolveToSignalObject=off  FilterRTWStateStorageClass=Auto  DifferentiatorICPrevScaledInput=0  DifferentiatorOutMin=[]  DifferentiatorOutMax=[]
  Id Controller1 : simulink/Continuous/PID Controller  Controller=PI  TimeDomain=Discrete-time  SampleTime=Ts  IntegratorMethod=Forward Euler  FilterMethod=Forward Euler  Form=Parallel  UseFilter=on  ControllerParametersSource=internal  P=0.1  I=0.01  D=0  N=100  InitialConditionSource=internal  InitialConditionForIntegrator=0  InitialConditionForFilter=0  ExternalReset=none  ZeroCross=off  LimitOutput=off  UpperSaturationLimit=2  LowerSaturationLimit=-2  LinearizeAsGain=off  AntiWindupMode=clamping  Kb=1  TrackingMode=off  Kt=1  PParamMin=[]  PParamMax=[]  IParamMin=[]  IParamMax=[]  DParamMin=[]  DParamMax=[]  NParamMin=[]  NParamMax=[]  KbParamMin=[]  KbParamMax=[]  KtParamMin=[]  KtParamMax=[]  POutMin=[]  POutMax=[]  IOutMin=[]  IOutMax=[]  DOutMin=[]  DOutMax=[]  NOutMin=[]  NOutMax=[]  KbOutMin=[]  KbOutMax=[]  KtOutMin=[]  KtOutMax=[]  IntegratorOutMin=[]  IntegratorOutMax=[]  FilterOutMin=[]  FilterOutMax=[]  SumOutMin=[]  SumOutMax=[]  SumI1OutMin=[]  SumI1OutMax=[]  SumI2OutMin=[]  SumI2OutMax=[]  SumI3OutMin=[]  SumI3OutMax=[]  SumDOutMin=[]  SumDOutMax=[]  SaturationOutMin=[]  SaturationOutMax=[]  IntegratorContinuousStateAttributes=''  IntegratorStateMustResolveToSignalObject=off  IntegratorRTWStateStorageClass=Auto  FilterContinuousStateAttributes=''  FilterStateMustResolveToSignalObject=off  FilterRTWStateStorageClass=Auto  DifferentiatorICPrevScaledInput=0  DifferentiatorOutMin=[]  DifferentiatorOutMax=[]
  K : Constant  Value=Vnom*2*sqrt(2/3)
  L : Gain  Gain=0.51311
  "L  " : Gain  Gain=0.51311
  L2 : Gain  Gain=-1
  Mux4 : Mux  Inputs=2
  Polar to Cartesian : simulink_extras/Transformations/Polar to Cartesian
  Product : Product  RndMeth=Zero
  Product1 : Product  RndMeth=Zero
  Product7 : Product  Inputs=**/  SaturateOnIntegerOverflow=on  InputSameDT=on  OutDataTypeStr=Inherit: Same as first input
  Saturation1 : Saturate  UpperLimit=inf  LowerLimit=-inf  SampleTime=Ts
  Saturation2 : Saturate  UpperLimit=inf  LowerLimit=-inf  SampleTime=Ts
  Scope1 : Scope  NumInputPorts=2
  Scope2 : Scope  NumInputPorts=2
  Scope3 : Scope  NumInputPorts=2
  Selector1 : Selector  InputPortWidth=2  IndexOptions=Index vector (dialog)  Indices=2  OutputSizes=[(-2)]
  Selector2 : Selector  InputPortWidth=2  IndexOptions=Index vector (dialog)  Indices=1  OutputSizes=[(-2)]
  Sum1 : Sum  Inputs=|+-  SaturateOnIntegerOverflow=on  InputSameDT=on  OutDataTypeStr=Inherit: Same as first input
  Sum2 : Sum  Inputs=|++  SaturateOnIntegerOverflow=on  InputSameDT=on  OutDataTypeStr=Inherit: Same as first input
  Sum3 : Sum  Inputs=|++  SaturateOnIntegerOverflow=on  InputSameDT=on  OutDataTypeStr=Inherit: Same as first input
  Sum4 : Sum  Inputs=|+-  SaturateOnIntegerOverflow=on  InputSameDT=on  OutDataTypeStr=Inherit: Same as first input
  "dq to ABC conversion " : Subsystem
  flux : Gain  Gain=-1/12
  flux1 : Bias  Bias=4
  flux2 : Gain  Gain=(Vnom*sqrt(3))/Pnom
  Uctrl_machine_conv : Outport
  wires:
  wr/1 -> [wr]
  " Vdq_s"/1 -> [Vdq]
  Idq_s/1 -> [Idq]
  Vdc_meas_V/1 -> [Vdc_V]
  r_angle_transform/1 -> [r_angle_transform]
  [Idq] -> Selector1/1
  Sum4/1 -> Id Controller1/1
  [Idq] -> Selector2/1
  Sum1/1 -> Id Controller/1
  Id Controller1/1 -> Sum2/1
  Id Controller/1 -> Sum3/1
  [wr] -> Product/1
  flux1/1 -> Product/2
  L/1 -> flux1/1
  "L  "/1 -> L2/1
  L2/1 -> Product1/1
  [wr] -> Product1/2
  Cartesian to Polar/1 -> Product7/1
  K/1 -> Product7/2
  Mux4/1 -> "dq to ABC conversion "/1(dq)  "Vdq0"
  Avoid division by zero/1 -> Product7/3
  [Vdc_V] -> Avoid division by zero/1
  Product7/1 -> 0-Mod_index_max_rotor/1  "m"
  Cartesian to Polar/2 -> Polar to Cartesian/2
  0-Mod_index_max_rotor/1 -> Polar to Cartesian/1
  Polar to Cartesian/1 -> Mux4/1
  Polar to Cartesian/2 -> Mux4/2
  Selector2/1 -> Feedback/1  "id"
  Feedback/1 -> Scope1/2, Sum1/2
  Feedback1/1 -> Scope2/2, Sum4/2
  Selector1/1 -> Feedback1/1  "iq"
  [r_angle_transform] -> "dq to ABC conversion "/2(Teta)
  "dq to ABC conversion "/1(ABC) -> Uctrl_machine_conv/1
  Sum3/1 -> Saturation2/1
  Saturation2/1 -> Scope3/1, Cartesian to Polar/1
  Sum2/1 -> Saturation1/1
  Saturation1/1 -> Scope3/2, Cartesian to Polar/2
  flux/1 -> flux2/1  "iq*"
  Feedback2/1 -> Scope2/1, Sum4/1
  Feedback3/1 -> Scope1/1, Sum1/1
  Fnom/1 -> Feedback3/1  "id*"
  Fnom1/1 -> L/1
  Tem_cmd/1 -> -2/1
  -2/1 -> flux/1
  flux2/1 -> Feedback2/1, "L  "/1

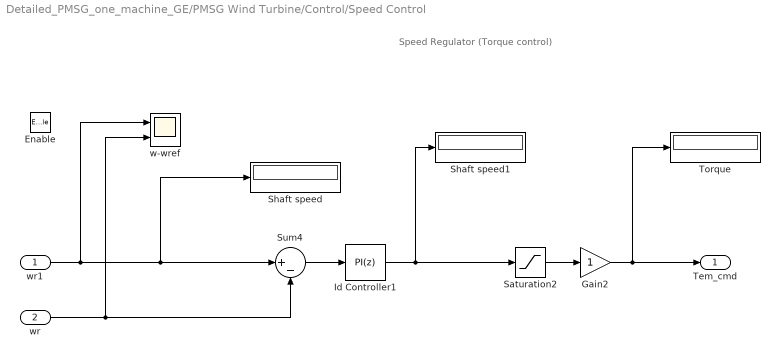
== system Detailed_PMSG_one_machine_GE/PMSG Wind Turbine/Control/Speed Control ==
  note: Speed Regulator
      | (Torque control)
  wr1 : Inport
  wr : Inport  Port=2
  Enable : EnablePort
  Gain2 : Gain  SampleTime=Ts
  Id Controller1 : simulink/Continuous/PID Controller  Controller=PI  TimeDomain=Discrete-time  SampleTime=Ts  IntegratorMethod=Forward Euler  FilterMethod=Forward Euler  Form=Parallel  UseFilter=on  ControllerParametersSource=internal  P=100  I=5  D=0  N=100  InitialConditionSource=internal  InitialConditionForIntegrator=0  InitialConditionForFilter=0  ExternalReset=none  ZeroCross=off  LimitOutput=off  UpperSaturationLimit=2  LowerSaturationLimit=-2  LinearizeAsGain=off  AntiWindupMode=clamping  Kb=1  TrackingMode=off  Kt=1  PParamMin=[]  PParamMax=[]  IParamMin=[]  IParamMax=[]  DParamMin=[]  DParamMax=[]  NParamMin=[]  NParamMax=[]  KbParamMin=[]  KbParamMax=[]  KtParamMin=[]  KtParamMax=[]  POutMin=[]  POutMax=[]  IOutMin=[]  IOutMax=[]  DOutMin=[]  DOutMax=[]  NOutMin=[]  NOutMax=[]  KbOutMin=[]  KbOutMax=[]  KtOutMin=[]  KtOutMax=[]  IntegratorOutMin=[]  IntegratorOutMax=[]  FilterOutMin=[]  FilterOutMax=[]  SumOutMin=[]  SumOutMax=[]  SumI1OutMin=[]  SumI1OutMax=[]  SumI2OutMin=[]  SumI2OutMax=[]  SumI3OutMin=[]  SumI3OutMax=[]  SumDOutMin=[]  SumDOutMax=[]  SaturationOutMin=[]  SaturationOutMax=[]  IntegratorContinuousStateAttributes=''  IntegratorStateMustResolveToSignalObject=off  IntegratorRTWStateStorageClass=Auto  FilterContinuousStateAttributes=''  FilterStateMustResolveToSignalObject=off  FilterRTWStateStorageClass=Auto  DifferentiatorICPrevScaledInput=0  DifferentiatorOutMin=[]  DifferentiatorOutMax=[]
  Saturation2 : Saturate  UpperLimit=0  LowerLimit=-1.1
  Shaft speed : Display
      settings: Decimation=1000
  Shaft speed1 : Display
      settings: Decimation=1000
  Sum4 : Sum  Inputs=|+-  SaturateOnIntegerOverflow=on  InputSameDT=on  OutDataTypeStr=Inherit: Same as first input
  Torque : Display
      settings: Decimation=1000
  w-wref : Scope  NumInputPorts=2
  Tem_cmd : Outport
  wires:
  Saturation2/1 -> Gain2/1
  Sum4/1 -> Id Controller1/1
  wr/1 -> w-wref/2, Sum4/2
  wr1/1 -> w-wref/1, Shaft speed/1, Sum4/1
  Id Controller1/1 -> Saturation2/1, Shaft speed1/1
  Gain2/1 -> Tem_cmd/1, Torque/1

== system Detailed_PMSG_one_machine_GE/PMSG Wind Turbine/pitch angle controller/pitch angle controller ==
  wg : Inport
  Ref : Inport  Port=2
  "0-pitch_max " : Saturate  UpperLimit=27  LowerLimit=0  SampleTime=Ts
  Discrete PID Controller : simulink/Continuous/PID Controller  Controller=P  TimeDomain=Discrete-time  SampleTime=Ts  IntegratorMethod=Forward Euler  FilterMethod=Forward Euler  Form=Parallel  UseFilter=on  ControllerParametersSource=internal  P=200  I=0  D=0  N=100  InitialConditionSource=internal  InitialConditionForIntegrator=0  InitialConditionForFilter=0  ExternalReset=none  ZeroCross=off  LimitOutput=on  UpperSaturationLimit=27  LowerSaturationLimit=0  LinearizeAsGain=off  AntiWindupMode=clamping  Kb=1  TrackingMode=off  Kt=1  PParamMin=[]  PParamMax=[]  IParamMin=[]  IParamMax=[]  DParamMin=[]  DParamMax=[]  NParamMin=[]  NParamMax=[]  KbParamMin=[]  KbParamMax=[]  KtParamMin=[]  KtParamMax=[]  POutMin=[]  POutMax=[]  IOutMin=[]  IOutMax=[]  DOutMin=[]  DOutMax=[]  NOutMin=[]  NOutMax=[]  KbOutMin=[]  KbOutMax=[]  KtOutMin=[]  KtOutMax=[]  IntegratorOutMin=[]  IntegratorOutMax=[]  FilterOutMin=[]  FilterOutMax=[]  SumOutMin=[]  SumOutMax=[]  SumI1OutMin=[]  SumI1OutMax=[]  SumI2OutMin=[]  SumI2OutMax=[]  SumI3OutMin=[]  SumI3OutMax=[]  SumDOutMin=[]  SumDOutMax=[]  SaturationOutMin=[]  SaturationOutMax=[]  IntegratorContinuousStateAttributes=''  IntegratorStateMustResolveToSignalObject=off  IntegratorRTWStateStorageClass=Auto  FilterContinuousStateAttributes=''  FilterStateMustResolveToSignalObject=off  FilterRTWStateStorageClass=Auto  DifferentiatorICPrevScaledInput=0  DifferentiatorOutMin=[]  DifferentiatorOutMax=[]
  Rate Limiter : RateLimiter  RisingSlewLimit=10  FallingSlewLimit=-10
  Sum3 : Sum  Inputs=|+-  SampleTime=Ts
  t=Pitch_time_constant1 : powerlib_extras/Discrete  Control Blocks/Discrete 1st-Order Filter  FilterType=Lowpass  Tc=0.02  Ts=Ts  Initialize=on  Vac_Init=[0.8 -25 60]*0  Vdc_Init=0  PlotResponse=off  param1=[1 500 0.1]
  pitch : Outport
  wires:
  Sum3/1 -> Discrete PID Controller/1
  wg/1 -> Sum3/1
  Ref/1 -> Sum3/2
  Rate Limiter/1 -> "0-pitch_max "/1
  "0-pitch_max "/1 -> t=Pitch_time_constant1/1
  t=Pitch_time_constant1/1 -> pitch/1
  Discrete PID Controller/1 -> Rate Limiter/1

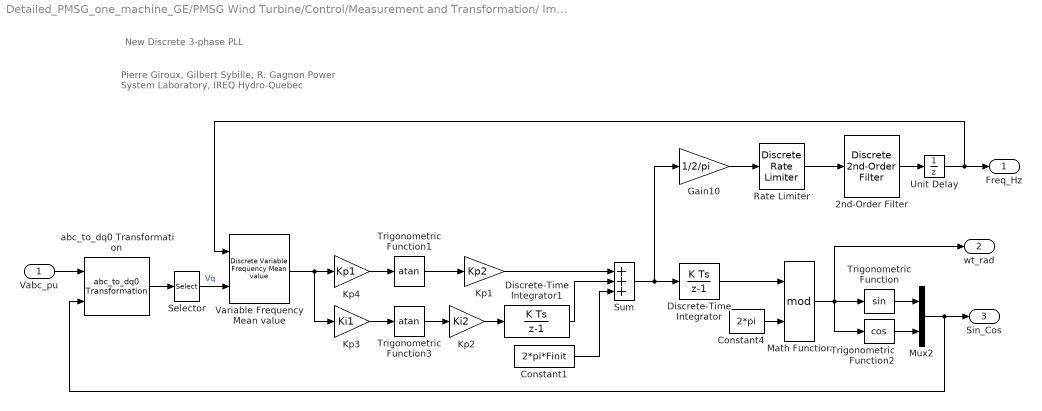
== system Detailed_PMSG_one_machine_GE/PMSG Wind Turbine/Control/Measurement and Transformation/ Improved Discrete 3-phase PLL ==
  note: New Discrete 3-phase PLL
  note: Pierre Giroux, Gilbert Sybille, R. Gagnon
      | Power System Laboratory, IREQ
      | Hydro-Quebec
  Vabc_pu : Inport  PortDimensions=3
  2nd-Order Filter : powerlib_extras/Discrete  Control Blocks/Discrete  2nd-Order Filter  FilterType=Lowpass  Fo=25  Zeta=0.707  Ts=Ts  Initialize=on  Vac_Init=[0 0 Finit]  Vdc_Init=Finit  PlotResponse=off  param1=[1 500 0.1]
  Constant1 : Constant  Value=2*pi*Finit
  Constant4 : Constant  Value=2*pi
  Discrete-Time Integrator : DiscreteIntegrator  SampleTime=Ts  ICPrevOutput=DiscIntNeverNeededParam  ICPrevScaledInput=DiscIntNeverNeededParam
  Discrete-Time Integrator1 : DiscreteIntegrator  gainval=1  SampleTime=Ts  LimitOutput=on  UpperSaturationLimit=2*pi*5  LowerSaturationLimit=-2*pi*5  ICPrevOutput=DiscIntNeverNeededParam  ICPrevScaledInput=DiscIntNeverNeededParam
  Gain10 : Gain  Gain=1/2/pi  SaturateOnIntegerOverflow=on  OutDataTypeStr=Inherit: Same as input  ParamDataTypeStr=Inherit: Same as input
  Kp1 : Gain  Gain=Kp2  SaturateOnIntegerOverflow=on  OutDataTypeStr=Inherit: Same as input  ParamDataTypeStr=Inherit: Same as input
  Kp2 : Gain  Gain=Ki2  SaturateOnIntegerOverflow=on  OutDataTypeStr=Inherit: Same as input  ParamDataTypeStr=Inherit: Same as input
  Kp3 : Gain  Gain=Ki1  SaturateOnIntegerOverflow=on  OutDataTypeStr=Inherit: Same as input  ParamDataTypeStr=Inherit: Same as input
  Kp4 : Gain  Gain=Kp1  SaturateOnIntegerOverflow=on  OutDataTypeStr=Inherit: Same as input  ParamDataTypeStr=Inherit: Same as input
  Math Function : Math  Operator=mod  SaturateOnIntegerOverflow=on
  Mux2 : Mux  Inputs=2
  Rate Limiter : powerlib_extras/Discrete  Control Blocks/Discrete Rate Limiter  R=12  F=-12  Vinit=Finit  Ts=Ts
  Selector : Selector  InputPortWidth=3  IndexOptions=Index vector (dialog)  Indices=2  OutputSizes=1
  Sum : Sum  Inputs=+++
  Trigonometric Function : Trigonometry
  Trigonometric Function1 : Trigonometry  Operator=atan
  Trigonometric Function2 : Trigonometry  Operator=cos
  Trigonometric Function3 : Trigonometry  Operator=atan
  Unit Delay : UnitDelay  InitialCondition=Finit  SampleTime=Ts
  Variable Frequency Mean value : powerlib_extras/Discrete Measurements/Discrete Variable Frequency Mean value  Finit=Finit  Fmin=Fmin  Vinit=0  Ts=Ts
  abc_to_dq0 Transformation : powerlib_extras/Measurements/abc_to_dq0 Transformation
  Freq_Hz : Outport
  wt_rad : Outport  Port=2
  Sin_Cos : Outport  Port=3
  wires:
  Vabc_pu/1 -> abc_to_dq0 Transformation/1
  abc_to_dq0 Transformation/1 -> Selector/1
  Constant4/1 -> Math Function/2
  Math Function/1 -> Trigonometric Function/1, Trigonometric Function2/1, wt_rad/1
  Trigonometric Function/1 -> Mux2/1
  Trigonometric Function2/1 -> Mux2/2
  Mux2/1 -> Sin_Cos/1, abc_to_dq0 Transformation/2
  Gain10/1 -> Rate Limiter/1
  Rate Limiter/1 -> 2nd-Order Filter/1
  2nd-Order Filter/1 -> Unit Delay/1
  Selector/1 -> Variable Frequency Mean value/2  "Vq"
  Kp4/1 -> Trigonometric Function1/1
  Trigonometric Function1/1 -> Kp1/1
  Constant1/1 -> Sum/3
  Variable Frequency Mean value/1 -> Kp4/1, Kp3/1
  Kp3/1 -> Trigonometric Function3/1
  Trigonometric Function3/1 -> Kp2/1
  Kp2/1 -> Discrete-Time Integrator1/1
  Sum/1 -> Discrete-Time Integrator/1, Gain10/1
  Unit Delay/1 -> Freq_Hz/1, Variable Frequency Mean value/1
  Discrete-Time Integrator/1 -> Math Function/1
  Kp1/1 -> Sum/1
  Discrete-Time Integrator1/1 -> Sum/2

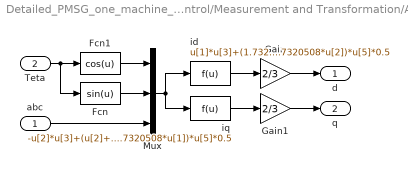
== system Detailed_PMSG_one_machine_GE/PMSG Wind Turbine/Control/Measurement and Transformation/ABC to dq conversion  ==
  abc : Inport
  Teta : Inport  Port=2
  Fcn : Fcn  Expr=sin(u)
  Fcn1 : Fcn  Expr=cos(u)
  Gain : Gain  Gain=2/3  SaturateOnIntegerOverflow=on  OutDataTypeStr=Inherit: Same as input  ParamDataTypeStr=Inherit: Same as input
  Gain1 : Gain  Gain=2/3  SaturateOnIntegerOverflow=on  OutDataTypeStr=Inherit: Same as input  ParamDataTypeStr=Inherit: Same as input
  Mux : Mux  Inputs=[1 1 3]
  id : Fcn  Expr=u[1]*u[3]+(1.7320508*u[2]-u[1])*u[4]*0.5+(-u[1]-1.7320508*u[2])*u[5]*0.5
  iq : Fcn  Expr=-u[2]*u[3]+(u[2]+1.7320508*u[1])*u[4]*0.5+(u[2]-1.7320508*u[1])*u[5]*0.5
  d : Outport  InitialOutput=0
  q : Outport  Port=2  InitialOutput=0
  wires:
  Fcn/1 -> Mux/2
  Fcn1/1 -> Mux/1
  Teta/1 -> Fcn1/1, Fcn/1
  Mux/1 -> iq/1, id/1
  abc/1 -> Mux/3
  iq/1 -> Gain1/1
  id/1 -> Gain/1
  Gain/1 -> d/1
  Gain1/1 -> q/1

== system Detailed_PMSG_one_machine_GE/PMSG Wind Turbine/Control/Measurement and Transformation/ABC to dq conversion ==
  abc : Inport
  Teta : Inport  Port=2
  Fcn : Fcn  Expr=sin(u)
  Fcn1 : Fcn  Expr=cos(u)
  Gain : Gain  Gain=2/3  SaturateOnIntegerOverflow=on  OutDataTypeStr=Inherit: Same as input  ParamDataTypeStr=Inherit: Same as input
  Gain1 : Gain  Gain=2/3  SaturateOnIntegerOverflow=on  OutDataTypeStr=Inherit: Same as input  ParamDataTypeStr=Inherit: Same as input
  Mux : Mux  Inputs=[1 1 3]
  id : Fcn  Expr=u[1]*u[3]+(1.7320508*u[2]-u[1])*u[4]*0.5+(-u[1]-1.7320508*u[2])*u[5]*0.5
  iq : Fcn  Expr=-u[2]*u[3]+(u[2]+1.7320508*u[1])*u[4]*0.5+(u[2]-1.7320508*u[1])*u[5]*0.5
  d : Outport  InitialOutput=0
  q : Outport  Port=2  InitialOutput=0
  wires:
  Fcn/1 -> Mux/2
  Fcn1/1 -> Mux/1
  Teta/1 -> Fcn1/1, Fcn/1
  Mux/1 -> iq/1, id/1
  abc/1 -> Mux/3
  iq/1 -> Gain1/1
  id/1 -> Gain/1
  Gain/1 -> d/1
  Gain1/1 -> q/1
